simulink model "heater_load"  (R2021a)
settings: Solver=VariableStepAuto  StartTime=0.0  StopTime=10.0  RelTol=1e-3
values from neighbouring files (symbols this model uses):
  c = 1005.4    [sldemo_househeat_data.m]
  cost = 0.09/3.6e6    (= 2.5e-08)    [sldemo_househeat_data.m]
  M = (lenHouse*widHouse*htHouse+tan(pitRoof)*widHouse*lenHouse)*densAir    [sldemo_househeat_data.m]
  Mdot = 3600    [sldemo_househeat_data.m]
  Req = RWall*RWindow/(RWall + RWindow)    [sldemo_househeat_data.m]
  THeater = 50    [sldemo_househeat_data.m]
  TinIC = 20    [sldemo_househeat_data.m]
libraries: simulink_extras x3
settings Model: Creator=hpirc  LastModifiedBy=hpirc

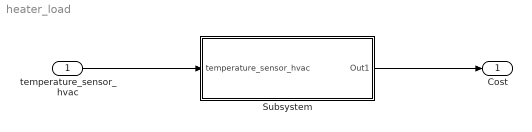
== system heater_load ==
  temperature_sensor_hvac : Inport
  Subsystem : Subsystem
  Cost : Outport
  wires:
  Subsystem/1(Out1) -> Cost/1
  temperature_sensor_hvac/1 -> Subsystem/1(temperature_sensor_hvac)

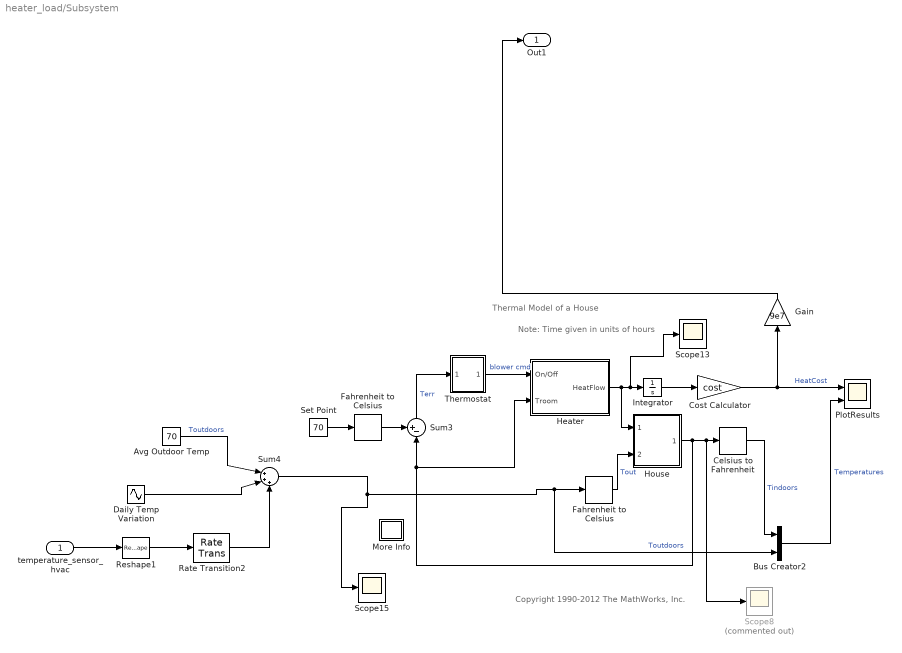
== system heater_load/Subsystem ==
  note: Copyright 1990-2012 The MathWorks, Inc.
  note: Thermal Model of a House
  note: Note: Time given in units of hours
  temperature_sensor_hvac : Inport
  Avg Outdoor Temp : Constant  Value=70
  Bus Creator2 : BusCreator  Inputs=2
  Celsius to Fahrenheit : simulink_extras/Transformations/Celsius to Fahrenheit
      settings: SourceProductBaseCode=SL
  Cost Calculator : Gain  Gain=cost  SaturateOnIntegerOverflow=on  OutDataTypeStr=Inherit: Same as input  ParamDataTypeStr=Inherit: Same as input
  Daily Temp Variation : Sin  Amplitude=-7  Frequency=2*pi/120  SampleTime=0
  Fahrenheit to Celsius : simulink_extras/Transformations/Fahrenheit to Celsius
      settings: SourceProductBaseCode=SL
  "Fahrenheit to Celsius " : simulink_extras/Transformations/Fahrenheit to Celsius
      settings: SourceProductBaseCode=SL
  Gain : Gain  Gain=9e7
  Heater : Subsystem
  House : Subsystem
      mask Display: image(fullfile(matlabroot,'toolbox','simulink','simdemos','simgeneral','images','HouseHeatHousePix.svg'))
  Integrator : Integrator  InitialCondition=TinIC
  More Info : Subsystem
      settings: OpenFcn=showExample('simulink_general/sldemo_househeatExample')
      mask Display: disp('?')
  PlotResults : Scope  NumInputPorts=2
  Rate Transition2 : RateTransition
  Reshape1 : Reshape
  Scope13 : Scope
  Scope15 : Scope
  Scope8 : Scope  Commented=on
  Set Point : Constant  Value=70
  Sum3 : Sum  Inputs=+-|  InputSameDT=on  SaturateOnIntegerOverflow=on  OutDataTypeStr=Inherit: Same as first input
  Sum4 : Sum  Inputs=|+++
  Thermostat : Subsystem
      mask Display: image(fullfile(matlabroot,'toolbox','simulink','simdemos','simgeneral','images','HouseHeatThermostatPix.svg'))
  Out1 : Outport
  wires:
  Fahrenheit to Celsius/1 -> House/2(Outdoor Temp Tout)  "Tout"
  Set Point/1 -> "Fahrenheit to Celsius "/1
  Cost Calculator/1 -> PlotResults/1, Gain/1  "HeatCost"
  Celsius to Fahrenheit/1 -> Bus Creator2/1  "Tindoors"
  Daily Temp Variation/1 -> Sum4/2
  Gain/1 -> Out1/1
  Avg Outdoor Temp/1 -> Sum4/1  "Toutdoors"
  Rate Transition2/1 -> Sum4/3
  Thermostat/1(Blower switch) -> Heater/1(On/Off)  "blower cmd"
  Bus Creator2/1 -> PlotResults/2  "Temperatures"
  "Fahrenheit to Celsius "/1 -> Sum3/1
  Sum3/1 -> Thermostat/1(Terr)  "Terr"
  temperature_sensor_hvac/1 -> Reshape1/1
  Heater/1(HeatFlow) -> Scope13/1, Integrator/1, House/1(Heater QDot In)
  Sum4/1 -> Scope15/1, Fahrenheit to Celsius/1, Bus Creator2/2  "Toutdoors"
  Integrator/1 -> Cost Calculator/1
  House/1(Room Temp Troom) -> Scope8/1, Celsius to Fahrenheit/1, Heater/2(Troom), Sum3/2
  Reshape1/1 -> Rate Transition2/1

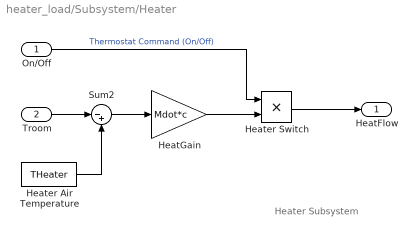
== system heater_load/Subsystem/Heater ==
  note: Heater Subsystem
  On/Off : Inport
  Troom : Inport  Port=2
  HeatGain : Gain  Gain=Mdot*c
  Heater Air Temperature : Constant  Value=THeater
  Heater Switch : Product  RndMeth=Zero
  Sum2 : Sum  Inputs=|-+
  HeatFlow : Outport  VectorParamsAs1DForOutWhenUnconnected=off
  wires:
  Heater Air Temperature/1 -> Sum2/2
  Troom/1 -> Sum2/1
  Sum2/1 -> HeatGain/1
  On/Off/1 -> Heater Switch/1  "Thermostat Command (On/Off)"
  HeatGain/1 -> Heater Switch/2
  Heater Switch/1 -> HeatFlow/1

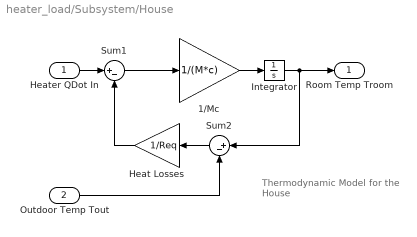
== system heater_load/Subsystem/House ==
  note: Thermodynamic Model
      | for the House
  Heater QDot In : Inport
  Outdoor Temp Tout : Inport  Port=2
  1/Mc : Gain  Gain=1/(M*c)  SaturateOnIntegerOverflow=on  OutDataTypeStr=Inherit: Same as input  ParamDataTypeStr=Inherit: Same as input
  Heat Losses : Gain  Gain=1/Req  SaturateOnIntegerOverflow=on  OutDataTypeStr=Inherit: Same as input  ParamDataTypeStr=Inherit: Same as input
  Integrator : Integrator  InitialCondition=TinIC
  Sum1 : Sum  Inputs=|+-  InputSameDT=on  SaturateOnIntegerOverflow=on  OutDataTypeStr=Inherit: Same as first input
  Sum2 : Sum  Inputs=|+-  InputSameDT=on  SaturateOnIntegerOverflow=on  OutDataTypeStr=Inherit: Same as first input
  Room Temp Troom : Outport  InitialOutput=0  VectorParamsAs1DForOutWhenUnconnected=off
  wires:
  Outdoor Temp Tout/1 -> Sum2/2
  Heater QDot In/1 -> Sum1/1
  Sum1/1 -> 1/Mc/1
  Sum2/1 -> Heat Losses/1
  Heat Losses/1 -> Sum1/2
  1/Mc/1 -> Integrator/1
  Integrator/1 -> Sum2/1, Room Temp Troom/1

== system heater_load/Subsystem/More Info ==

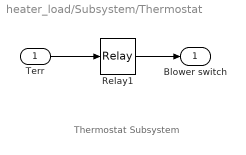
== system heater_load/Subsystem/Thermostat ==
  note: Thermostat Subsystem
  Terr : Inport
  Relay1 : Relay  OnSwitchValue=5*(5/9)  OffSwitchValue=-5*(5/9)
  Blower switch : Outport  InitialOutput=0  VectorParamsAs1DForOutWhenUnconnected=off
  wires:
  Terr/1 -> Relay1/1
  Relay1/1 -> Blower switch/1
